simulink library "TemperatureSwitch"  (R2016b)
settings: Solver=VariableStepAuto  StartTime=0.0  StopTime=10.0  RelTol=1e-3
settings Model: Creator=Marc  LastModifiedBy=Marc

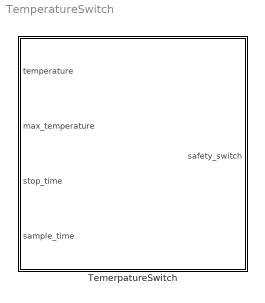
== system TemperatureSwitch ==
  TemerpatureSwitch : Subsystem

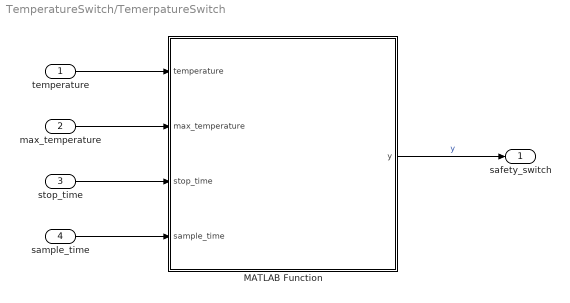
== system TemperatureSwitch/TemerpatureSwitch ==
  "temperature " : Inport
  max_temperature : Inport  Port=2
  stop_time : Inport  Port=3
  sample_time : Inport  Port=4
  MATLAB Function : MATLAB Function  TreatAsAtomicUnit=on
  safety_switch : Outport
  wires:
  MATLAB Function/1(y) -> safety_switch/1  "y"
  "temperature "/1 -> MATLAB Function/1(temperature)
  sample_time/1 -> MATLAB Function/4(sample_time)
  stop_time/1 -> MATLAB Function/3(stop_time)
  max_temperature/1 -> MATLAB Function/2(max_temperature)

== matlab function TemperatureSwitch/TemerpatureSwitch/MATLAB Function ==
  data: temperature input; y output; max_temperature input; stop_time input; sample_time input
function y = func_temperature_switch(temperature,max_temperature, stop_time, sample_time)

    persistent time_out
    
    if (isempty(time_out))
        time_out = 0;               % temperature is 'measured' every half second to check change over time
    end
            
    %sets output to true if temperature exceeds max temperature
    if temperature > max_temperature 
        y = true;
        
        time_out = stop_time/sample_time; %ensures a full stop for 60seconds once limits are exceeded
        
        %keeps quick stop activated for the intended 60 seconds during time out
    elseif time_out > 0
        y = true;        
    else
        % if noting is wrong keeps somanet on
        y = false;      
    end
    
    %counts down 
    if time_out ~=0
        time_out = time_out  - 1;
    end


end
